simulink subsystem "State_Machine_S1"  (R2023b)
settings: Solver=VariableStepAuto  StartTime=0.0  StopTime=10.0  RelTol=1e-3
settings Model: Creator=Inver  LastModifiedBy=Inver

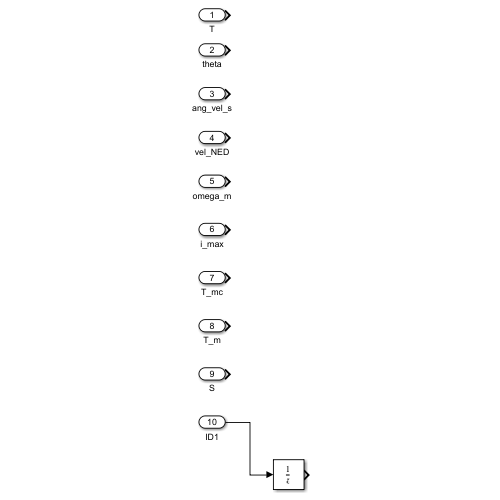
[thumbnail: Simulink's stored preview of the top-level diagram]
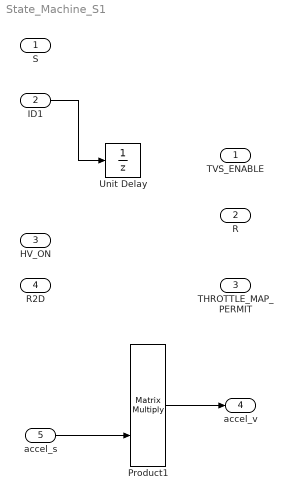
== system State_Machine_S1 ==
  S : Inport
  ID1 : Inport  Port=2
  HV_ON : Inport  Port=3
  R2D : Inport  Port=4
  accel_s : Inport  Port=5
  Product1 : Product  Multiplication=Matrix(*)
  Unit Delay : UnitDelay  SampleTime=-1  HasFrameUpgradeWarning=on
  TVS_ENABLE : Outport
  R : Outport  Port=2
  THROTTLE_MAP_PERMIT : Outport  Port=3
  accel_v : Outport  Port=4
  wires:
  ID1/1 -> Unit Delay/1
  Product1/1 -> accel_v/1
  accel_s/1 -> Product1/2
